simulink model "flash_led"  (R2026a)
settings: Solver=FixedStepDiscrete  StopTime=0.5
model workspace (MAT data in the model file):
  MAX_COUNT = 5000000
libraries: hdlsllib x1
settings Model: DataTypeOverride=Off  Creator=KoayXianCong  LastModifiedBy=KoayXianCong
settings OptimizationCC: ConditionallyExecuteInputs=off  InheritOutputTypeSmallerThanSingle=on
settings DebuggingCC: ArtificialAlgebraicLoopMsg=error  SingleTaskRateTransMsg=error
settings HardwareCC: ProdHWDeviceType=ASIC/FPGA->ASIC/FPGA  TargetBitPerPointer=64.0  TargetBitPerSizeT=64.0  TargetBitPerPtrDiffT=64.0  TargetLongLongMode=on  TargetIntDivRoundTo=Zero  TargetEndianess=LittleEndian  TargetWordSize=64.0  TargetHWDeviceType=Custom Processor->MATLAB Host Computer  ProdEqTarget=off

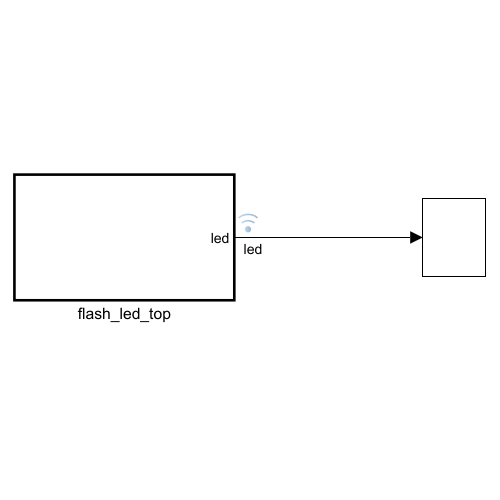
[thumbnail: Simulink's stored preview of the top-level diagram]
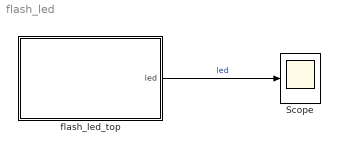
== system flash_led ==
  Scope : Scope
      settings: ActiveDisplayYMinimum=-14.874999999999996  ActiveDisplayYMaximum=143.875
  flash_led_top : Subsystem  TreatAsAtomicUnit=on
  wires:
  flash_led_top/1(led) -> Scope/1  "led"

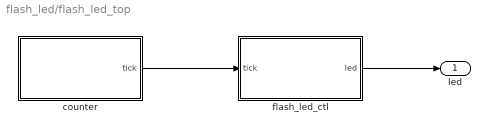
== system flash_led/flash_led_top ==
  counter : Subsystem
  flash_led_ctl : Subsystem
  led : Outport
  wires:
  counter/1(tick) -> flash_led_ctl/1(tick)
  flash_led_ctl/1(led) -> led/1

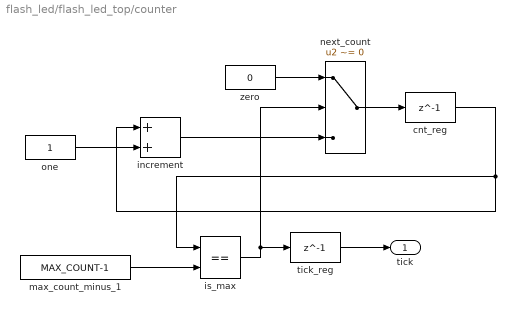
== system flash_led/flash_led_top/counter ==
  cnt_reg : Delay  DelayLength=1  InitialCondition=0
  increment : Sum  OutDataTypeStr=fixdt(0,23,0)
  is_max : RelationalOperator  Operator===  OutDataTypeStr=boolean
  max_count_minus_1 : Constant  Value=MAX_COUNT-1  OutDataTypeStr=fixdt(0,23,0)
  next_count : Switch  Criteria=u2 ~= 0
  one : Constant  OutDataTypeStr=fixdt(0,23,0)
  tick_reg : Delay  DelayLength=1  InitialCondition=0
  zero : Constant  Value=0  OutDataTypeStr=fixdt(0,23,0)
  tick : Outport
  wires:
  cnt_reg/1 -> increment/1, is_max/1
  one/1 -> increment/2
  max_count_minus_1/1 -> is_max/2
  zero/1 -> next_count/1
  is_max/1 -> next_count/2, tick_reg/1
  increment/1 -> next_count/3
  next_count/1 -> cnt_reg/1
  tick_reg/1 -> tick/1

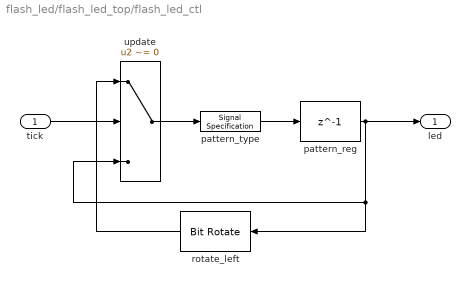
== system flash_led/flash_led_top/flash_led_ctl ==
  tick : Inport
  pattern_reg : Delay  DelayLength=1  InitialCondition=1
  pattern_type : SignalSpecification  OutDataTypeStr=uint8
  rotate_left : hdlsllib/Logic and Bit Operations/Bit Rotate  mode=Rotate Left  N=1
  update : Switch  Criteria=u2 ~= 0
  led : Outport
  wires:
  tick/1 -> update/2
  update/1 -> pattern_type/1
  pattern_type/1 -> pattern_reg/1
  pattern_reg/1 -> rotate_left/1, update/3, led/1
  rotate_left/1 -> update/1
